simulink model "sistemi_me_vonese_fikse"  (R2016b)
settings: Solver=VariableStepAuto  StartTime=0.0  StopTime=20  RelTol=1e-3
libraries: simulink x1
settings Model: Creator=aidbu  LastModifiedBy=aidbu

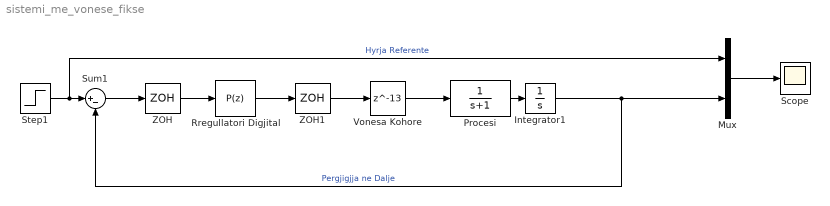
== system sistemi_me_vonese_fikse ==
  Integrator1 : Integrator
  Mux : Mux  Inputs=2
  Procesi : TransferFcn  Denominator=[1 1]
  Rregullatori Digjital : simulink/Continuous/PID Controller  Controller=P  TimeDomain=Discrete-time  SampleTime=0.1  IntegratorMethod=Forward Euler  FilterMethod=Forward Euler  Form=Parallel  UseFilter=on  ControllerParametersSource=internal  P=0.5377  I=1  D=0  N=100  InitialConditionSource=internal  InitialConditionForIntegrator=0  InitialConditionForFilter=0  ExternalReset=none  LimitOutput=off  UpperSaturationLimit=inf  LowerSaturationLimit=-inf  LinearizeAsGain=off  AntiWindupMode=none  Kb=1  TrackingMode=off  Kt=1  PParamMin=[]  PParamMax=[]  IParamMin=[]  IParamMax=[]  DParamMin=[]  DParamMax=[]  NParamMin=[]  NParamMax=[]  KbParamMin=[]  KbParamMax=[]  KtParamMin=[]  KtParamMax=[]  POutMin=[]  POutMax=[]  IOutMin=[]  IOutMax=[]  DOutMin=[]  DOutMax=[]  NOutMin=[]  NOutMax=[]  KbOutMin=[]  KbOutMax=[]  KtOutMin=[]  KtOutMax=[]  IntegratorOutMin=[]  IntegratorOutMax=[]  FilterOutMin=[]  FilterOutMax=[]  SumOutMin=[]  SumOutMax=[]  SumI1OutMin=[]  SumI1OutMax=[]  SumI2OutMin=[]  SumI2OutMax=[]  SumI3OutMin=[]  SumI3OutMax=[]  SumDOutMin=[]  SumDOutMax=[]  SaturationOutMin=[]  SaturationOutMax=[]  IntegratorContinuousStateAttributes=''  IntegratorStateMustResolveToSignalObject=off  IntegratorRTWStateStorageClass=Auto  FilterContinuousStateAttributes=''  FilterStateMustResolveToSignalObject=off  FilterRTWStateStorageClass=Auto  DifferentiatorICPrevScaledInput=0  DifferentiatorOutMin=[]  DifferentiatorOutMax=[]
  Scope : Scope
  Step1 : Step  Time=0  SampleTime=0
  Sum1 : Sum  Inputs=|+-
  Vonesa Kohore : Delay  DelayLength=13  SampleTime=0.1
  ZOH : ZeroOrderHold  SampleTime=0.1
  ZOH1 : ZeroOrderHold  SampleTime=0.1
  wires:
  Procesi/1 -> Integrator1/1
  Step1/1 -> Mux/1, Sum1/1  "Hyrja Referente"
  Sum1/1 -> ZOH/1
  ZOH/1 -> Rregullatori Digjital/1
  Rregullatori Digjital/1 -> ZOH1/1
  Integrator1/1 -> Sum1/2, Mux/2  "Pergjigjja ne Dalje"
  ZOH1/1 -> Vonesa Kohore/1
  Vonesa Kohore/1 -> Procesi/1
  Mux/1 -> Scope/1
